simulink model "eVTOL_PX4_2023b"  (R2024b)
settings: Solver=ode4  StartTime=0  StopTime=inf  FixedStep=0.01  RelTol=1e-3
values from neighbouring files (symbols this model uses):
  aDl =     [initdata.mat]
  aDr =     [initdata.mat]
  aDyn =     [initdata.mat]
  Airport = init_airport('PHNL')    [initdata_HIL_eVTOL.m]
  aLat =     [initdata.mat]
  aLon =     [initdata.mat]
  D = Prop.D    [EOM_dt_MC.m]    (also in EOM_get_alf_dt_de_prop_evtol.m = CD * QS)
  dt0 = X(2)    [EOM_get_alf_dt_de_prop_evtol.m]    (also in initdata.mat = 0.258252593971; initdata_HIL_eVTOL.m = EOM_dt_MC)
  EAS0 = TAS0 / EAS2TAS    [initdata_HIL_eVTOL.m]
  FCS = init_FCS    [initdata_HIL_eVTOL.m]
  General = init_layoutdata    [EOM_dt_MC.m]    (also in build_optimized_CA.m; initdata.mat = ; initdata_HIL_eVTOL.m)
  h0 = Con(1)    [EOM_get_alf_dt_de_prop_evtol.m]    (also in initdata.mat = 450; initdata_HIL_eVTOL.m = 50)
  mass = Con(3)    [EOM_get_alf_dt_de_prop_evtol.m]    (also in initdata.mat = 2255.54; initdata_HIL_eVTOL.m = 7)
  Motor = init_motor_evtol    [EOM_dt_MC.m]    (also in initdata.mat = []; initdata_HIL_eVTOL.m)
  Prop = init_propeller_evtol_new    [EOM_dt_MC.m]    (also in initdata_HIL_eVTOL.m)
  R2D = 180/pi    (= 57.2957795131)    [EOM_get_alf_dt_de_prop_evtol.m]    (also in init_FCS.m; init_aerodata_evtol.m; init_airport.m; initdata.mat)
  SAMPLE_TIME = 0.01    [initdata_HIL_eVTOL.m]
  theta0 = -0.0510981441662    [initdata.mat]
undefined symbols (not defined in the file or in its folder): A1, aDa, aDe, aero, asbhl20env, B1, C1, de0, Earth, Environment, INIT_Data, InitData, Kd, Kp, magnitude, Newton, pProp, Raphson, Tc, WGS84
libraries: simulink_extras x63, vrlib x48, sharedtransform x28, simulink x22, slpidlib x20, sharedutil x20, matrix_library x18, aerolibwindfilters x12, aerolibobsolete x8, aerolibasang x8, aerolibatmos2 x6, aerolibfltsims x6
(part 9 of 17)

== system eVTOL_PX4_2023b/Subsystem1/Energy & Power1/thrust_5/Propeller  ==
  rpm : Inport
  V : Inport  Port=2
  rho : Inport  Port=3
  D^5 : Constant  Value=5
  Diameter : Constant  Value=Prop.D
  Divide : Product  Inputs=4
  Divide2 : Product  Inputs=4
  Divide3 : Product  Inputs=**/
  Gain : Gain  Gain=1/60
  Math Function : Math  Operator=magnitude^2  SignedPower=on
  Math Function1 : Math  Operator=magnitude^2  SignedPower=on
  Math Function2 : Math  Operator=magnitude^2  SignedPower=on
  Math Function3 : Math  Operator=pow  SignedPower=on
  Math Function4 : Math  Operator=pow  SignedPower=on
  Scope{,1..4} (5 alike) : Scope
  Subsystem : Subsystem
  get CP : Lookup_n-D  BreakpointsForDimension1=Prop.J  BreakpointsForDimension2=Prop.rpm_grid  IndexSearchMethod=Linear search  BeginIndexSearchUsingPreviousIndexResult=on  Table=Prop.CP  RndMeth=Simplest
      settings: InputPortMap=u0,u1
  get CT : Lookup_n-D  BreakpointsForDimension1=Prop.J  BreakpointsForDimension2=Prop.rpm_grid  IndexSearchMethod=Linear search  BeginIndexSearchUsingPreviousIndexResult=on  Table=Prop.CT  RndMeth=Simplest
      settings: InputPortMap=u0,u1
  "n^3 " : Constant  Value=3
  P_plr (w) : Outport  VectorParamsAs1DForOutWhenUnconnected=off
  T (N) : Outport  Port=2  VectorParamsAs1DForOutWhenUnconnected=off
  eta_p : Outport  Port=3  VectorParamsAs1DForOutWhenUnconnected=off
  wires:
  Divide2/1 -> P_plr (w)/1, Scope/1
  Divide3/1 -> eta_p/1  "eta_p"
  D^5/1 -> Math Function4/2
  Math Function4/1 -> Divide2/4
  "n^3 "/1 -> Math Function3/2
  Math Function3/1 -> Divide2/3
  get CP/1 -> Divide3/3, Divide2/1, Scope3/1
  Subsystem/1(J) -> Scope2/1, get CT/1, Divide3/1, get CP/1
  Divide/1 -> Scope1/1, T (N)/1
  Math Function2/1 -> Divide/4  "D^4"
  Math Function1/1 -> Math Function2/1
  Diameter/1 -> Math Function1/1, Math Function4/1
  Math Function/1 -> Divide/3  "n^2"
  Gain/1 -> Math Function3/1, Math Function/1
  rho/1 -> Divide/2, Divide2/2
  get CT/1 -> Divide3/2, Divide/1, Scope4/1
  V/1 -> Subsystem/1(V)
  rpm/1 -> get CP/2, get CT/2, Gain/1, Subsystem/2(rpm)

== system eVTOL_PX4_2023b/Subsystem1/Energy & Power1/thrust_6/Motor ==
  P_shaft : Inport
  dt : Inport  Port=2
  V : Inport  Port=3
  rpm0 : Inport  Port=4
  rho : Inport  Port=5
  rpm_grid : Inport  Port=6
  Constant : Constant  Value=Motor.Ue
  Constant1 : Constant  Value=Motor.Re
  Constant2 : Constant  Value=Motor.Rm
  Constant3 : Constant  Value=Motor.KE
  Constant4 : Constant  Value=Motor.KT  VectorParams1D=off
  Constant5 : Constant  Value=Motor.Im0
  Constant6 : Constant  Value=0
  D^5 : Constant  Value=5
  Diameter : Constant  Value=Prop.D
  Diameter1 : Constant  Value=Prop.D
  Divide : Product  Inputs=*//
  Ea : Sum  Inputs=+-
  Gain1 : Gain  Gain=30/pi
  Gain2 : Gain  Gain=pi/30
  Gain3 : Gain  Gain=1/60
  Gain4 : Gain  Gain=1/(2*pi)
  Im : Sum
  Integrator : Integrator  InitialConditionSource=external  InitialCondition=600
  Ix : Constant  Value=Prop.Ix
  J : Product  Inputs=*//
  Manual Switch : ManualSwitch
  Math Function : Math  Operator=magnitude^2  SignedPower=on
  Math Function3 : Math  Operator=pow  SignedPower=on
  Math Function4 : Math  Operator=pow  SignedPower=on
  Memory : Memory  InitialCondition=0.1
  N(rpm) : Product  Inputs=*/
  N(rpm)1 : Product  Inputs=/*
  P Scope : Scope  NumInputPorts=2
  P_sp : Product  Inputs=4
  Product1 : Product
  Product2 : Product
  Q : Product  Inputs=4
  RPM 6 : Scope
  Saturation : Saturate  UpperLimit=1047.2  LowerLimit=0.1
  Scope : Scope
  Sum : Sum  Inputs=|+-
  Ueo : Product
  Um : Sum  Inputs=+-
  get CP : Lookup_n-D  BreakpointsForDimension1=Prop.J  BreakpointsForDimension2=Prop.rpm_grid  IndexSearchMethod=Linear search  BeginIndexSearchUsingPreviousIndexResult=on  Table=Prop.CP  RndMeth=Simplest
      settings: InputPortMap=u0,u1
  "n^3 " : Constant  Value=3
  rpm : Outport  VectorParamsAs1DForOutWhenUnconnected=off
  wires:
  Saturation/1 -> Gain1/1, Divide/2
  Gain2/1 -> Integrator/2
  rpm0/1 -> Manual Switch/1
  Gain1/1 -> rpm/1, RPM 6/1  "rpm"
  Sum/1 -> Divide/1  "DP"
  Divide/1 -> Integrator/1  "omega_dot"
  dt/1 -> Ueo/1
  Integrator/1 -> Saturation/1  "omega"
  P_sp/1 -> Scope/1, P Scope/1, Sum/1
  P_shaft/1 -> P Scope/2, Sum/2
  Ix/1 -> Divide/3
  Constant/1 -> Ueo/2
  Ueo/1 -> Um/1
  Product1/1 -> Um/2
  Constant1/1 -> Product1/1
  Um/1 -> Ea/1
  Product2/1 -> Ea/2
  Constant2/1 -> Product2/1
  Ea/1 -> N(rpm)/1
  Constant3/1 -> N(rpm)/2
  Diameter/1 -> J/2
  V/1 -> J/1
  N(rpm)/1 -> Gain3/1
  J/1 -> get CP/1
  rpm_grid/1 -> get CP/2
  Gain4/1 -> Q/2  "CQ"
  D^5/1 -> Math Function4/2
  Diameter1/1 -> Math Function4/1
  Math Function/1 -> Q/3  "n^2"
  Q/1 -> N(rpm)1/2
  Constant4/1 -> N(rpm)1/1
  N(rpm)1/1 -> Im/1
  Constant5/1 -> Im/2
  Im/1 -> Product1/2, Product2/2
  rho/1 -> Q/1, P_sp/3  "rho"
  Math Function3/1 -> P_sp/2  "n^3"
  "n^3 "/1 -> Math Function3/2
  Math Function4/1 -> Q/4, P_sp/4  "D^5"
  get CP/1 -> Gain4/1, P_sp/1  "CP"
  Constant6/1 -> Manual Switch/2
  Manual Switch/1 -> Gain2/1
  Gain3/1 -> Memory/1  "rps"
  Memory/1 -> J/3, Math Function3/1, Math Function/1

== system eVTOL_PX4_2023b/Subsystem1/Energy & Power1/thrust_6/Propeller  ==
  rpm : Inport
  V : Inport  Port=2
  rho : Inport  Port=3
  D^5 : Constant  Value=5
  Diameter : Constant  Value=Prop.D
  Divide : Product  Inputs=4
  Divide2 : Product  Inputs=4
  Divide3 : Product  Inputs=**/
  Gain : Gain  Gain=1/60
  Math Function : Math  Operator=magnitude^2  SignedPower=on
  Math Function1 : Math  Operator=magnitude^2  SignedPower=on
  Math Function2 : Math  Operator=magnitude^2  SignedPower=on
  Math Function3 : Math  Operator=pow  SignedPower=on
  Math Function4 : Math  Operator=pow  SignedPower=on
  Scope{,1..4} (5 alike) : Scope
  Subsystem : Subsystem
  get CP : Lookup_n-D  BreakpointsForDimension1=Prop.J  BreakpointsForDimension2=Prop.rpm_grid  IndexSearchMethod=Linear search  BeginIndexSearchUsingPreviousIndexResult=on  Table=Prop.CP  RndMeth=Simplest
      settings: InputPortMap=u0,u1
  get CT : Lookup_n-D  BreakpointsForDimension1=Prop.J  BreakpointsForDimension2=Prop.rpm_grid  IndexSearchMethod=Linear search  BeginIndexSearchUsingPreviousIndexResult=on  Table=Prop.CT  RndMeth=Simplest
      settings: InputPortMap=u0,u1
  "n^3 " : Constant  Value=3
  P_plr (w) : Outport  VectorParamsAs1DForOutWhenUnconnected=off
  T (N) : Outport  Port=2  VectorParamsAs1DForOutWhenUnconnected=off
  eta_p : Outport  Port=3  VectorParamsAs1DForOutWhenUnconnected=off
  wires:
  Divide2/1 -> P_plr (w)/1, Scope/1
  Divide3/1 -> eta_p/1  "eta_p"
  D^5/1 -> Math Function4/2
  Math Function4/1 -> Divide2/4
  "n^3 "/1 -> Math Function3/2
  Math Function3/1 -> Divide2/3
  get CP/1 -> Divide3/3, Divide2/1, Scope3/1
  Subsystem/1(J) -> Scope2/1, get CT/1, Divide3/1, get CP/1
  Divide/1 -> Scope1/1, T (N)/1
  Math Function2/1 -> Divide/4  "D^4"
  Math Function1/1 -> Math Function2/1
  Diameter/1 -> Math Function1/1, Math Function4/1
  Math Function/1 -> Divide/3  "n^2"
  Gain/1 -> Math Function3/1, Math Function/1
  rho/1 -> Divide/2, Divide2/2
  get CT/1 -> Divide3/2, Divide/1, Scope4/1
  V/1 -> Subsystem/1(V)
  rpm/1 -> get CP/2, get CT/2, Gain/1, Subsystem/2(rpm)

== system eVTOL_PX4_2023b/Subsystem1/Environment/Wind Models/Dryden Wind Turbulence Model (Continuous (+q -r)) ==
  Altitude : Inport  Unit=m
  Airspeed : Inport  Port=2  Unit=m/s
  DCM : Inport  Port=3  Unit=1  PortDimensions=[3 3]
  (u,v,w) : Selector  InputPortWidth=4  IndexOptions=Index vector (dialog)  Indices=[1 2 3]  OutputSizes=1
  Angle Conversion : Subsystem
  Bus Creator : BusCreator  Inputs=3
  Cast : DataTypeConversion  SaturateOnIntegerOverflow=off  RndMeth=Floor
  Cast To Double{,1..4} (5 alike) : DataTypeConversion  OutDataTypeStr=double  SaturateOnIntegerOverflow=off  RndMeth=Floor
  Disallow CGS : UnitConfiguration  UnitSystemsStr=English,SI,SI (extended)  AllowAllUnitSystems=off
  Filters on angular rates : Subsystem  mask(Angular Rates){}
  Filters on velocities : aerolibwindfilters/Dryden Continuous Filters  SystemSampleTime=-1  VariantActivationTime=update diagram  AllowFlexibleInterface=on  Latency=0  AutoFrameSizeCalculation=off
  Length Conversion : Subsystem
  Length Conversion1 : Subsystem
  Mux : Mux  Inputs=3
  Mux1 : Mux  Inputs=3
  RMS turbulence intensities : Subsystem
  Select angular rates : Subsystem
  Select velocities : Subsystem
  Turbulence scale lengths : Subsystem
  Unit Conversion : UnitConversion  OutputType=Inherit: Inherit via back propagation
  Velocity Conversion : Subsystem
  Velocity Conversion2 : Subsystem
  White Noise : aerolibcommonsys/Tunable White Noise  pwr=[1 1 1 1]*pi  Ts=ts  seed=Seed
  Wind direction : Constant  Value=Wdeg
  Windspeed at 20ft (6m) : Constant  Value=W20
  Wingspan : Constant  Value=Wingspan
  p : Selector  InputPortWidth=4  IndexOptions=Index vector (dialog)  Indices=[4]  OutputSizes=1
  ug,vg,wg : Outport  Unit=m/s  VectorParamsAs1DForOutWhenUnconnected=off
  pg,qg,rg : Outport  Port=2  VectorParamsAs1DForOutWhenUnconnected=off
  wires:
  Cast To Double4/1 -> Velocity Conversion/1(in)
  Airspeed/1 -> Cast To Double4/1
  Cast To Double3/1 -> Length Conversion1/1(in)
  Wingspan/1 -> Cast To Double3/1
  Cast To Double2/1 -> Length Conversion/1(in)
  Cast To Double1/1 -> Angle Conversion/1(in)
  Cast To Double/1 -> Bus Creator/1  "DCM"
  Mux1/1 -> Cast/1
  Cast/1 -> pg,qg,rg/1
  (u,v,w)/1 -> Filters on velocities/1
  Unit Conversion/1 -> ug,vg,wg/1
  Velocity Conversion/1(out) -> Filters on angular rates/3(V), Filters on velocities/8
  Angle Conversion/1(out) -> Bus Creator/2  "Wdeg"
  Length Conversion1/1(out) -> Filters on angular rates/7(wingspan)
  Bus Creator/1 -> Select angular rates/4("DCM, altitude, Wdeg"), Select velocities/1("DCM, altitude, Wdeg")
  DCM/1 -> Cast To Double/1  "DCM"
  Wind direction/1 -> Cast To Double1/1
  Select angular rates/3(rgw) -> Mux1/3
  Select angular rates/2(qgw) -> Mux1/2
  Select angular rates/1(pgw) -> Mux1/1
  Select velocities/3(wgw) -> Mux/3
  Select velocities/2(vgw) -> Mux/2
  Select velocities/1(ugw) -> Mux/1
  Velocity Conversion2/1(out) -> RMS turbulence intensities/2(Windspeed at 20ft (6m))
  Windspeed at 20ft (6m)/1 -> Velocity Conversion2/1(in)
  RMS turbulence intensities/2(sigma_vg) -> Filters on velocities/6
  Filters on velocities/3 -> Filters on angular rates/2(wg), Select velocities/4(wgw_h&l)  "wgw"
  Filters on velocities/2 -> Filters on angular rates/1(vg), Select velocities/3(vgw_h&l)  "vgw"
  RMS turbulence intensities/1("sigma_ug ") -> Filters on velocities/5
  Filters on velocities/1 -> Select velocities/2(ugw_h&l)  "ugw"
  Filters on angular rates/3(rgw) -> Select angular rates/3(rgw_h&l)  "rgw"
  Filters on angular rates/2(qgw) -> Select angular rates/2(qgw_h&l)  "qgw"
  Filters on angular rates/1(pgw) -> Select angular rates/1(pgw_h&l)  "pgw"
  RMS turbulence intensities/3(sigma_wg) -> Filters on angular rates/5(sigma_w), Filters on velocities/7
  Turbulence scale lengths/3(L_wg) -> Filters on angular rates/4(Lw), Filters on velocities/4
  Turbulence scale lengths/1(L_ug) -> Filters on velocities/2
  Altitude/1 -> Cast To Double2/1
  Mux/1 -> Unit Conversion/1
  White Noise/1 -> (u,v,w)/1, p/1
  p/1 -> Filters on angular rates/6(Noise)
  Length Conversion/1(out) -> Bus Creator/3, RMS turbulence intensities/1(Altitude), Turbulence scale lengths/1(Altitude)  "altitude"
  Turbulence scale lengths/2(L_vg) -> Filters on velocities/3

== system eVTOL_PX4_2023b/Subsystem1/Environment1/Wind Models/Dryden Wind Turbulence Model (Continuous (+q -r)) ==
  Altitude : Inport  Unit=m
  Airspeed : Inport  Port=2  Unit=m/s
  DCM : Inport  Port=3  Unit=1  PortDimensions=[3 3]
  (u,v,w) : Selector  InputPortWidth=4  IndexOptions=Index vector (dialog)  Indices=[1 2 3]  OutputSizes=1
  Angle Conversion : Subsystem
  Bus Creator : BusCreator  Inputs=3
  Cast : DataTypeConversion  SaturateOnIntegerOverflow=off  RndMeth=Floor
  Cast To Double{,1..4} (5 alike) : DataTypeConversion  OutDataTypeStr=double  SaturateOnIntegerOverflow=off  RndMeth=Floor
  Disallow CGS : UnitConfiguration  UnitSystemsStr=English,SI,SI (extended)  AllowAllUnitSystems=off
  Filters on angular rates : Subsystem  mask(Angular Rates){}
  Filters on velocities : aerolibwindfilters/Dryden Continuous Filters  SystemSampleTime=-1  VariantActivationTime=update diagram  AllowFlexibleInterface=on  Latency=0  AutoFrameSizeCalculation=off
  Length Conversion : Subsystem
  Length Conversion1 : Subsystem
  Mux : Mux  Inputs=3
  Mux1 : Mux  Inputs=3
  RMS turbulence intensities : Subsystem
  Select angular rates : Subsystem
  Select velocities : Subsystem
  Turbulence scale lengths : Subsystem
  Unit Conversion : UnitConversion  OutputType=Inherit: Inherit via back propagation
  Velocity Conversion : Subsystem
  Velocity Conversion2 : Subsystem
  White Noise : aerolibcommonsys/Tunable White Noise  pwr=[1 1 1 1]*pi  Ts=ts  seed=Seed
  Wind direction : Constant  Value=Wdeg
  Windspeed at 20ft (6m) : Constant  Value=W20
  Wingspan : Constant  Value=Wingspan
  p : Selector  InputPortWidth=4  IndexOptions=Index vector (dialog)  Indices=[4]  OutputSizes=1
  ug,vg,wg : Outport  Unit=m/s  VectorParamsAs1DForOutWhenUnconnected=off
  pg,qg,rg : Outport  Port=2  VectorParamsAs1DForOutWhenUnconnected=off
  wires:
  Cast To Double4/1 -> Velocity Conversion/1(in)
  Airspeed/1 -> Cast To Double4/1
  Cast To Double3/1 -> Length Conversion1/1(in)
  Wingspan/1 -> Cast To Double3/1
  Cast To Double2/1 -> Length Conversion/1(in)
  Cast To Double1/1 -> Angle Conversion/1(in)
  Cast To Double/1 -> Bus Creator/1  "DCM"
  Mux1/1 -> Cast/1
  Cast/1 -> pg,qg,rg/1
  (u,v,w)/1 -> Filters on velocities/1
  Unit Conversion/1 -> ug,vg,wg/1
  Velocity Conversion/1(out) -> Filters on angular rates/3(V), Filters on velocities/8
  Angle Conversion/1(out) -> Bus Creator/2  "Wdeg"
  Length Conversion1/1(out) -> Filters on angular rates/7(wingspan)
  Bus Creator/1 -> Select angular rates/4("DCM, altitude, Wdeg"), Select velocities/1("DCM, altitude, Wdeg")
  DCM/1 -> Cast To Double/1  "DCM"
  Wind direction/1 -> Cast To Double1/1
  Select angular rates/3(rgw) -> Mux1/3
  Select angular rates/2(qgw) -> Mux1/2
  Select angular rates/1(pgw) -> Mux1/1
  Select velocities/3(wgw) -> Mux/3
  Select velocities/2(vgw) -> Mux/2
  Select velocities/1(ugw) -> Mux/1
  Velocity Conversion2/1(out) -> RMS turbulence intensities/2(Windspeed at 20ft (6m))
  Windspeed at 20ft (6m)/1 -> Velocity Conversion2/1(in)
  RMS turbulence intensities/2(sigma_vg) -> Filters on velocities/6
  Filters on velocities/3 -> Filters on angular rates/2(wg), Select velocities/4(wgw_h&l)  "wgw"
  Filters on velocities/2 -> Filters on angular rates/1(vg), Select velocities/3(vgw_h&l)  "vgw"
  RMS turbulence intensities/1("sigma_ug ") -> Filters on velocities/5
  Filters on velocities/1 -> Select velocities/2(ugw_h&l)  "ugw"
  Filters on angular rates/3(rgw) -> Select angular rates/3(rgw_h&l)  "rgw"
  Filters on angular rates/2(qgw) -> Select angular rates/2(qgw_h&l)  "qgw"
  Filters on angular rates/1(pgw) -> Select angular rates/1(pgw_h&l)  "pgw"
  RMS turbulence intensities/3(sigma_wg) -> Filters on angular rates/5(sigma_w), Filters on velocities/7
  Turbulence scale lengths/3(L_wg) -> Filters on angular rates/4(Lw), Filters on velocities/4
  Turbulence scale lengths/1(L_ug) -> Filters on velocities/2
  Altitude/1 -> Cast To Double2/1
  Mux/1 -> Unit Conversion/1
  White Noise/1 -> (u,v,w)/1, p/1
  p/1 -> Filters on angular rates/6(Noise)
  Length Conversion/1(out) -> Bus Creator/3, RMS turbulence intensities/1(Altitude), Turbulence scale lengths/1(Altitude)  "altitude"
  Turbulence scale lengths/2(L_vg) -> Filters on velocities/3

== system eVTOL_PX4_2023b/Subsystem1/airframe/Flight Conditions/Incidence, Sideslip, & Airspeed ==
  Vb : Inport
  Airspeed : Math  Operator=sqrt  SignedPower=on
  Incidence : Trigonometry  Operator=atan2
  Product : Product  Inputs=*/  SaturateOnIntegerOverflow=on  OutDataTypeStr=Inherit: Same as first input
  Sideslip : Trigonometry  Operator=asin
  Subsystem : Subsystem
  Subsystem1 : Subsystem
  dot : Subsystem
  Alpha : Outport  InitialOutput=0  VectorParamsAs1DForOutWhenUnconnected=off
  Beta : Outport  Port=2  InitialOutput=0  VectorParamsAs1DForOutWhenUnconnected=off
  V : Outport  Port=3  InitialOutput=0  VectorParamsAs1DForOutWhenUnconnected=off
  wires:
  Product/1 -> Sideslip/1
  Subsystem/1(w) -> Incidence/1
  Subsystem/2(U) -> Incidence/2
  dot/1(dot) -> Airspeed/1
  Airspeed/1 -> Product/2, V/1
  Incidence/1 -> Alpha/1
  Vb/1 -> Subsystem/1(V), dot/1(Vb), Subsystem1/1(V)
  Sideslip/1 -> Beta/1
  Subsystem1/1(v) -> Product/1

== system eVTOL_PX4_2023b/Subsystem1/airframe/Flight Conditions/Subsystem ==
  <Ve> : Inport
  Atan1 : Trigonometry  Operator=atan2
  Atan2 : Trigonometry  Operator=atan2
  Dot Product : DotProduct  OutDataTypeStr=Inherit: Inherit via internal rule
  Gain : Gain  Gain=-1
  Selector : Selector  InputPortWidth=3  IndexOptions=Index vector (dialog)  Indices=1  OutputSizes=1
  Selector1 : Selector  InputPortWidth=3  IndexOptions=Index vector (dialog)  Indices=2  OutputSizes=1
  Selector2 : Selector  InputPortWidth=3  IndexOptions=Index vector (dialog)  Indices=3  OutputSizes=1
  Sqrt : Sqrt
  gamma : Outport  InitialOutput=0  VectorParamsAs1DForOutWhenUnconnected=off
  chi : Outport  Port=2  InitialOutput=0  VectorParamsAs1DForOutWhenUnconnected=off
  V : Outport  Port=3  InitialOutput=0  VectorParamsAs1DForOutWhenUnconnected=off
  wires:
  Selector/1 -> Atan1/2
  Selector2/1 -> Gain/1
  <Ve>/1 -> Selector/1, Selector1/1, Selector2/1, Dot Product/1, Dot Product/2
  Atan2/1 -> gamma/1
  Selector1/1 -> Atan1/1
  Sqrt/1 -> V/1, Atan2/2
  Atan1/1 -> chi/1
  Gain/1 -> Atan2/1
  Dot Product/1 -> Sqrt/1

== system eVTOL_PX4_2023b/Subsystem1/airframe/force moment/Gear&FM in body axis ==
  PlantData : Inport
  Add1 : Sum  Inputs=++++
  Add2 : Sum  Inputs=++++
  Constant1 : Constant  Value=0
  Constant6 : Constant  Value=0
  F 4 gear : Scope  NumInputPorts=4
  F&M  Front Gear Left : Subsystem
  F&M  Front Gear Right : Subsystem
  F&M  Main Gear Left : Subsystem
  F&M  Main Gear Right : Subsystem
  M 4 gear : Scope  NumInputPorts=4
  F_Gear : Outport  VectorParamsAs1DForOutWhenUnconnected=off
  M_Gear : Outport  Port=2  VectorParamsAs1DForOutWhenUnconnected=off
  wires:
  PlantData/1 -> F&M  Main Gear Right/1(PlantData), F&M  Main Gear Left/1(PlantData), F&M  Front Gear Right/1(PlantData), F&M  Front Gear Left/1(PlantData)
  F&M  Front Gear Left/2(M_fgl) -> M 4 gear/1, Add2/1
  F&M  Front Gear Left/1(F_fgl) -> F 4 gear/1, Add1/1
  F&M  Front Gear Right/1(F_fgl) -> F 4 gear/2, Add1/2
  F&M  Main Gear Left/1(F_fgl) -> F 4 gear/3, Add1/3
  F&M  Main Gear Right/1(F_fgl) -> F 4 gear/4, Add1/4
  Add1/1 -> F_Gear/1
  F&M  Front Gear Right/2(M_fgl) -> M 4 gear/2, Add2/2
  F&M  Main Gear Left/2(M_fgl) -> M 4 gear/3, Add2/3
  F&M  Main Gear Right/2(M_fgl) -> M 4 gear/4, Add2/4
  Add2/1 -> M_Gear/1
  Constant6/1 -> F&M  Main Gear Left/2(dg)
  Constant1/1 -> F&M  Main Gear Right/2(dg)

== system eVTOL_PX4_2023b/Subsystem1/airframe/force moment/Gear&FM in body axis1 ==
  PlantData : Inport
  Add1 : Sum  Inputs=++++
  Add2 : Sum  Inputs=++++
  Constant1 : Constant  Value=0
  Constant6 : Constant  Value=0
  F 4 gear : Scope  NumInputPorts=4
  F&M  Front Gear Left : Subsystem
  F&M  Front Gear Right : Subsystem
  F&M  Main Gear Left : Subsystem
  F&M  Main Gear Right : Subsystem
  M 4 gear : Scope  NumInputPorts=4
  F_Gear : Outport  VectorParamsAs1DForOutWhenUnconnected=off
  M_Gear : Outport  Port=2  VectorParamsAs1DForOutWhenUnconnected=off
  wires:
  PlantData/1 -> F&M  Main Gear Right/1(PlantData), F&M  Main Gear Left/1(PlantData), F&M  Front Gear Right/1(PlantData), F&M  Front Gear Left/1(PlantData)
  F&M  Front Gear Left/2(M_fgl) -> M 4 gear/1, Add2/1
  F&M  Front Gear Left/1(F_fgl) -> F 4 gear/1, Add1/1
  F&M  Front Gear Right/1(F_fgl) -> F 4 gear/2, Add1/2
  F&M  Main Gear Left/1(F_fgl) -> F 4 gear/3, Add1/3
  F&M  Main Gear Right/1(F_fgl) -> F 4 gear/4, Add1/4
  Add1/1 -> F_Gear/1
  F&M  Front Gear Right/2(M_fgl) -> M 4 gear/2, Add2/2
  F&M  Main Gear Left/2(M_fgl) -> M 4 gear/3, Add2/3
  F&M  Main Gear Right/2(M_fgl) -> M 4 gear/4, Add2/4
  Add2/1 -> M_Gear/1
  Constant6/1 -> F&M  Main Gear Left/2(dg)
  Constant1/1 -> F&M  Main Gear Right/2(dg)

== system eVTOL_PX4_2023b/Subsystem1/airframe/force moment/Thrust&M in body axis ==
  prop : Inport
  3x3 Cross Product{,1..5} (6 alike) : sharedutil/3x3 Cross Product  aMode=aMode
  Bus Selector1 : BusSelector  OutputSignals=T_1,T_2,T_3,T_4,T_5,T_6,Q
  Constant1 : Constant  Value=General.pos_plr3
  Constant2 : Constant  Value=General.pos_plr4
  Constant3 : Constant  Value=General.pos_plr5
  Constant4 : Constant  Value=General.pos_plr1
  Constant5 : Constant  Value=General.pos_plr6
  Constant6 : Constant  Value=General.pos_plr2
  Display3 : Display
  Scope2 : Scope
  Sum2 : Sum  Inputs=++++++
  Sum3 : Sum  Inputs=++++++
  Sum4 : Sum  Inputs=++|
  T MC : Scope  NumInputPorts=6
  f_T : Outport  VectorParamsAs1DForOutWhenUnconnected=off
  m_T : Outport  Port=2  VectorParamsAs1DForOutWhenUnconnected=off
  wires:
  prop/1 -> Bus Selector1/1
  Constant4/1 -> 3x3 Cross Product/1
  Constant6/1 -> 3x3 Cross Product1/1
  Constant1/1 -> 3x3 Cross Product2/1
  Constant2/1 -> 3x3 Cross Product3/1
  Bus Selector1/1 -> T MC/1, [T_1]  "<T_1>"
  Bus Selector1/2 -> [T_2], T MC/2  "<T_2>"
  Bus Selector1/3 -> [T_3], T MC/3  "<T_3>"
  Bus Selector1/4 -> [T_4], T MC/4  "<T_4>"
  [T_1] -> 3x3 Cross Product/2
  [T_2] -> 3x3 Cross Product1/2
  [T_3] -> 3x3 Cross Product2/2
  [T_4] -> 3x3 Cross Product3/2
  [T_1] -> Sum2/1
  [T_2] -> Sum2/2
  [T_3] -> Sum2/3
  [T_4] -> Sum2/4
  3x3 Cross Product/1 -> Sum3/1
  3x3 Cross Product1/1 -> Sum3/2
  3x3 Cross Product2/1 -> Sum3/3
  3x3 Cross Product3/1 -> Sum3/4
  Sum2/1 -> f_T/1, Scope2/1, Display3/1  "T"
  Sum3/1 -> Sum4/2
  Bus Selector1/5 -> [T_5], T MC/5  "<T_5>"
  Sum4/1 -> m_T/1
  [Q] -> Sum4/1
  Bus Selector1/6 -> T MC/6, [T_6]  "<T_6>"
  Bus Selector1/7 -> [Q]  "<Q>"
  [T_5] -> Sum2/5
  [T_6] -> Sum2/6
  [T_5] -> 3x3 Cross Product4/2
  3x3 Cross Product4/1 -> Sum3/5
  Constant3/1 -> 3x3 Cross Product4/1
  [T_6] -> 3x3 Cross Product5/2
  3x3 Cross Product5/1 -> Sum3/6
  Constant5/1 -> 3x3 Cross Product5/1

== system eVTOL_PX4_2023b/Subsystem1/airframe/force moment/aero F&M in body axis ==
  PlantData : Inport
  Act_surface : Inport  Port=2
  Aerodynamic Coefficients : Subsystem  AncestorBlock=asbhl20vehicle/Vehicle/Aerodynamic/Aerodynamic Coefficients
      settings: LibrarySourceBlock=|
      | asbhl20vehicle/Vehicle/Aerodynamic/Aerodynamic
      | Coefficients
  "Aerodynamic Forces and Moments " : aerolibadyn/Aerodynamic Forces and Moments   inputAxes=Body  outputForceAxes=Body  outputMomentAxes=Body  S=General.Sw  b=General.b  cbar=General.MAC
  Center of Gravity : Constant  Value=[0 0 0]  SampleTime=0
  Center of Pressure : Constant  Value=[0 0 0]  SampleTime=0
  Constant : Constant
  Constant1 : Constant  Commented=on
  Mux1 : Mux  Inputs=2
  PlantBus : BusSelector  OutputSignals=Vb,alpha,beta,Va,pqr,alphaDot,mach
  PlantBus1 : BusSelector  OutputSignals=Q
  PlantData_1 : InportShadow
  Product : Product
  Product1 : Product
  Scope1 : Scope  Commented=on
  Scope2 : Scope
  Scope3 : Scope
  Scope4 : Scope  Commented=on
  Selector : Selector  Commented=on  InputPortWidth=3  IndexOptions=Index vector (dialog)  Indices=1  OutputSizes=1
  Switch : Switch  Commented=on  Criteria=u2 > Threshold  Threshold=3  SaturateOnIntegerOverflow=off  InputSameDT=off
  nonunit value : Subsystem
  Fb (X Y Z) : Outport  VectorParamsAs1DForOutWhenUnconnected=off
  M (L M N) : Outport  Port=2  VectorParamsAs1DForOutWhenUnconnected=off
  wires:
  "Aerodynamic Forces and Moments "/1 -> Product/1, Scope2/1
  "Aerodynamic Forces and Moments "/2 -> Product1/1, Scope3/1
  PlantData/1 -> PlantBus/1
  Act_surface/1 -> Aerodynamic Coefficients/5(Act_surface)
  PlantBus/2 -> Mux1/1  "<alpha>"
  PlantBus/3 -> Mux1/2  "<beta>"
  PlantBus/5 -> nonunit value/2(pqr)  "<pqr>"
  Center of Gravity/1 -> "Aerodynamic Forces and Moments "/3
  Center of Pressure/1 -> "Aerodynamic Forces and Moments "/4
  PlantBus1/1 -> "Aerodynamic Forces and Moments "/2  "<Q>"
  PlantData_1/1 -> PlantBus1/1
  PlantBus/6 -> nonunit value/3(alphaDot)  "<alphaDot>"
  PlantBus/4 -> nonunit value/1(V)  "<Va>"
  Constant1/1 -> Switch/1
  Constant/1 -> [Aero_SW]
  Switch/1 -> Scope1/1
  Product/1 -> Fb (X Y Z)/1
  Product1/1 -> M (L M N)/1
  [Aero_SW] -> Product/2
  [Aero_SW] -> Product1/2
  PlantBus/1 -> Selector/1  "<Vb>"
  Selector/1 -> Switch/2, Scope4/1  "Vb_x"
  Mux1/1 -> Aerodynamic Coefficients/1(Incid)
  nonunit value/1(pqr_n) -> Aerodynamic Coefficients/3(pqrn)
  nonunit value/2(alphaDot_n) -> Aerodynamic Coefficients/4(alphaDot_n)
  Aerodynamic Coefficients/1(Coeff) -> "Aerodynamic Forces and Moments "/1
  PlantBus/7 -> Aerodynamic Coefficients/2(mach)  "<mach>"

== system eVTOL_PX4_2023b/Subsystem1/airframe/force moment/gravity in body axis ==
  PlantData : Inport
  EnvmData : Inport  Port=2
  Bus Selector1 : BusSelector  OutputSignals=DCM_be,mass
  Bus Selector2 : BusSelector  OutputSignals=g
  G in body axis : Product  Multiplication=Matrix(*)  RndMeth=Zero
  Gain1 : Gain  Gain=[0; 0; 1]
  Product : Product  RndMeth=Zero
  Fb : Outport  VectorParamsAs1DForOutWhenUnconnected=off
  wires:
  Bus Selector1/1 -> G in body axis/1  "<DCM_be>"
  Gain1/1 -> G in body axis/2
  Bus Selector1/2 -> Product/1  "<mass>"
  Bus Selector2/1 -> Product/2  "<g>"
  Product/1 -> Gain1/1  "mg"
  PlantData/1 -> Bus Selector1/1
  G in body axis/1 -> Fb/1
  EnvmData/1 -> Bus Selector2/1

== system eVTOL_PX4_2023b/Subsystem1/airframe1/Flight Conditions/Incidence, Sideslip, & Airspeed ==
  Vb : Inport
  Airspeed : Math  Operator=sqrt  SignedPower=on
  Incidence : Trigonometry  Operator=atan2
  Product : Product  Inputs=*/  SaturateOnIntegerOverflow=on  OutDataTypeStr=Inherit: Same as first input
  Sideslip : Trigonometry  Operator=asin
  Subsystem : Subsystem
  Subsystem1 : Subsystem
  dot : Subsystem
  Alpha : Outport  InitialOutput=0  VectorParamsAs1DForOutWhenUnconnected=off
  Beta : Outport  Port=2  InitialOutput=0  VectorParamsAs1DForOutWhenUnconnected=off
  V : Outport  Port=3  InitialOutput=0  VectorParamsAs1DForOutWhenUnconnected=off
  wires:
  Product/1 -> Sideslip/1
  Subsystem/1(w) -> Incidence/1
  Subsystem/2(U) -> Incidence/2
  dot/1(dot) -> Airspeed/1
  Airspeed/1 -> Product/2, V/1
  Incidence/1 -> Alpha/1
  Vb/1 -> Subsystem/1(V), dot/1(Vb), Subsystem1/1(V)
  Sideslip/1 -> Beta/1
  Subsystem1/1(v) -> Product/1

== system eVTOL_PX4_2023b/Subsystem1/airframe1/Flight Conditions/Subsystem ==
  <Ve> : Inport
  Atan1 : Trigonometry  Operator=atan2
  Atan2 : Trigonometry  Operator=atan2
  Dot Product : DotProduct  OutDataTypeStr=Inherit: Inherit via internal rule
  Gain : Gain  Gain=-1
  Selector : Selector  InputPortWidth=3  IndexOptions=Index vector (dialog)  Indices=1  OutputSizes=1
  Selector1 : Selector  InputPortWidth=3  IndexOptions=Index vector (dialog)  Indices=2  OutputSizes=1
  Selector2 : Selector  InputPortWidth=3  IndexOptions=Index vector (dialog)  Indices=3  OutputSizes=1
  Sqrt : Sqrt
  gamma : Outport  InitialOutput=0  VectorParamsAs1DForOutWhenUnconnected=off
  chi : Outport  Port=2  InitialOutput=0  VectorParamsAs1DForOutWhenUnconnected=off
  V : Outport  Port=3  InitialOutput=0  VectorParamsAs1DForOutWhenUnconnected=off
  wires:
  Selector/1 -> Atan1/2
  Selector2/1 -> Gain/1
  <Ve>/1 -> Selector/1, Selector1/1, Selector2/1, Dot Product/1, Dot Product/2
  Atan2/1 -> gamma/1
  Selector1/1 -> Atan1/1
  Sqrt/1 -> V/1, Atan2/2
  Atan1/1 -> chi/1
  Gain/1 -> Atan2/1
  Dot Product/1 -> Sqrt/1

== system eVTOL_PX4_2023b/Subsystem1/airframe1/force moment/Gear&FM in body axis ==
  PlantData : Inport
  Add1 : Sum  Inputs=++++
  Add2 : Sum  Inputs=++++
  Constant1 : Constant  Value=0
  Constant6 : Constant  Value=0
  F 4 gear : Scope  NumInputPorts=4
  F&M  Front Gear Left : Subsystem
  F&M  Front Gear Right : Subsystem
  F&M  Main Gear Left : Subsystem
  F&M  Main Gear Right : Subsystem
  M 4 gear : Scope  NumInputPorts=4
  F_Gear : Outport  VectorParamsAs1DForOutWhenUnconnected=off
  M_Gear : Outport  Port=2  VectorParamsAs1DForOutWhenUnconnected=off
  wires:
  PlantData/1 -> F&M  Main Gear Right/1(PlantData), F&M  Main Gear Left/1(PlantData), F&M  Front Gear Right/1(PlantData), F&M  Front Gear Left/1(PlantData)
  F&M  Front Gear Left/2(M_fgl) -> M 4 gear/1, Add2/1
  F&M  Front Gear Left/1(F_fgl) -> F 4 gear/1, Add1/1
  F&M  Front Gear Right/1(F_fgl) -> F 4 gear/2, Add1/2
  F&M  Main Gear Left/1(F_fgl) -> F 4 gear/3, Add1/3
  F&M  Main Gear Right/1(F_fgl) -> F 4 gear/4, Add1/4
  Add1/1 -> F_Gear/1
  F&M  Front Gear Right/2(M_fgl) -> M 4 gear/2, Add2/2
  F&M  Main Gear Left/2(M_fgl) -> M 4 gear/3, Add2/3
  F&M  Main Gear Right/2(M_fgl) -> M 4 gear/4, Add2/4
  Add2/1 -> M_Gear/1
  Constant6/1 -> F&M  Main Gear Left/2(dg)
  Constant1/1 -> F&M  Main Gear Right/2(dg)

== system eVTOL_PX4_2023b/Subsystem1/airframe1/force moment/Gear&FM in body axis1 ==
  PlantData : Inport
  Add1 : Sum  Inputs=++++
  Add2 : Sum  Inputs=++++
  Constant1 : Constant  Value=0
  Constant6 : Constant  Value=0
  F 4 gear : Scope  NumInputPorts=4
  F&M  Front Gear Left : Subsystem
  F&M  Front Gear Right : Subsystem
  F&M  Main Gear Left : Subsystem
  F&M  Main Gear Right : Subsystem
  Gain : Gain  Gain=0.005
  Gain1 : Gain  Gain=0.005
  M 4 gear : Scope  NumInputPorts=4
  F_Gear : Outport  VectorParamsAs1DForOutWhenUnconnected=off
  M_Gear : Outport  Port=2  VectorParamsAs1DForOutWhenUnconnected=off
  wires:
  PlantData/1 -> F&M  Main Gear Right/1(PlantData), F&M  Main Gear Left/1(PlantData), F&M  Front Gear Right/1(PlantData), F&M  Front Gear Left/1(PlantData)
  F&M  Front Gear Left/2(M_fgl) -> M 4 gear/1, Add2/1
  F&M  Front Gear Left/1(F_fgl) -> F 4 gear/1, Add1/1
  F&M  Front Gear Right/1(F_fgl) -> F 4 gear/2, Add1/2
  F&M  Main Gear Left/1(F_fgl) -> F 4 gear/3, Add1/3
  F&M  Main Gear Right/1(F_fgl) -> F 4 gear/4, Add1/4
  F&M  Front Gear Right/2(M_fgl) -> M 4 gear/2, Add2/2
  F&M  Main Gear Left/2(M_fgl) -> M 4 gear/3, Add2/3
  F&M  Main Gear Right/2(M_fgl) -> M 4 gear/4, Add2/4
  Constant6/1 -> F&M  Main Gear Left/2(dg)
  Constant1/1 -> F&M  Main Gear Right/2(dg)
  Add1/1 -> Gain/1
  Gain/1 -> F_Gear/1
  Add2/1 -> Gain1/1
  Gain1/1 -> M_Gear/1

== system eVTOL_PX4_2023b/Subsystem1/airframe1/force moment/Thrust&M in body axis ==
  prop : Inport
  3x3 Cross Product{,1..5} (6 alike) : sharedutil/3x3 Cross Product  aMode=aMode
  Bus Selector1 : BusSelector  OutputSignals=T_1,T_2,T_3,T_4,T_5,T_6,Q
  Constant1 : Constant  Value=General.pos_plr3
  Constant2 : Constant  Value=General.pos_plr4
  Constant3 : Constant  Value=General.pos_plr5
  Constant4 : Constant  Value=General.pos_plr1
  Constant5 : Constant  Value=General.pos_plr6
  Constant6 : Constant  Value=General.pos_plr2
  Display3 : Display
  Scope2 : Scope
  Sum2 : Sum  Inputs=++++++
  Sum3 : Sum  Inputs=++++++
  Sum4 : Sum  Inputs=++|
  T MC : Scope  NumInputPorts=6
  f_T : Outport  VectorParamsAs1DForOutWhenUnconnected=off
  m_T : Outport  Port=2  VectorParamsAs1DForOutWhenUnconnected=off
  wires:
  prop/1 -> Bus Selector1/1
  Constant4/1 -> 3x3 Cross Product/1
  Constant6/1 -> 3x3 Cross Product1/1
  Constant1/1 -> 3x3 Cross Product2/1
  Constant2/1 -> 3x3 Cross Product3/1
  Bus Selector1/1 -> T MC/1, [T_1]  "<T_1>"
  Bus Selector1/2 -> [T_2], T MC/2  "<T_2>"
  Bus Selector1/3 -> [T_3], T MC/3  "<T_3>"
  Bus Selector1/4 -> [T_4], T MC/4  "<T_4>"
  [T_1] -> 3x3 Cross Product/2
  [T_2] -> 3x3 Cross Product1/2
  [T_3] -> 3x3 Cross Product2/2
  [T_4] -> 3x3 Cross Product3/2
  [T_1] -> Sum2/1
  [T_2] -> Sum2/2
  [T_3] -> Sum2/3
  [T_4] -> Sum2/4
  3x3 Cross Product/1 -> Sum3/1
  3x3 Cross Product1/1 -> Sum3/2
  3x3 Cross Product2/1 -> Sum3/3
  3x3 Cross Product3/1 -> Sum3/4
  Sum2/1 -> f_T/1, Scope2/1, Display3/1  "T"
  Sum3/1 -> Sum4/2
  Bus Selector1/5 -> [T_5], T MC/5  "<T_5>"
  Sum4/1 -> m_T/1
  [Q] -> Sum4/1
  Bus Selector1/6 -> T MC/6, [T_6]  "<T_6>"
  Bus Selector1/7 -> [Q]  "<Q>"
  [T_5] -> Sum2/5
  [T_6] -> Sum2/6
  [T_5] -> 3x3 Cross Product4/2
  3x3 Cross Product4/1 -> Sum3/5
  Constant3/1 -> 3x3 Cross Product4/1
  [T_6] -> 3x3 Cross Product5/2
  3x3 Cross Product5/1 -> Sum3/6
  Constant5/1 -> 3x3 Cross Product5/1

== system eVTOL_PX4_2023b/Subsystem1/airframe1/force moment/aero F&M in body axis ==
  PlantData : Inport
  Act_surface : Inport  Port=2
  Aerodynamic Coefficients : Subsystem  AncestorBlock=asbhl20vehicle/Vehicle/Aerodynamic/Aerodynamic Coefficients
      settings: LibrarySourceBlock=|
      | asbhl20vehicle/Vehicle/Aerodynamic/Aerodynamic
      | Coefficients
  "Aerodynamic Forces and Moments " : aerolibadyn/Aerodynamic Forces and Moments   inputAxes=Body  outputForceAxes=Body  outputMomentAxes=Body  S=General.Sw  b=General.b  cbar=General.MAC
  Center of Gravity : Constant  Value=[0 0 0]  SampleTime=0
  Center of Pressure : Constant  Value=[0 0 0]  SampleTime=0
  Constant : Constant
  Constant1 : Constant  Commented=on
  Mux1 : Mux  Inputs=2
  PlantBus : BusSelector  OutputSignals=Vb,alpha,beta,Va,pqr,alphaDot,mach
  PlantBus1 : BusSelector  OutputSignals=Q
  PlantData_1 : InportShadow
  Product : Product
  Product1 : Product
  Scope1 : Scope  Commented=on
  Scope2 : Scope
  Scope3 : Scope
  Scope4 : Scope  Commented=on
  Selector : Selector  Commented=on  InputPortWidth=3  IndexOptions=Index vector (dialog)  Indices=1  OutputSizes=1
  Switch : Switch  Commented=on  Criteria=u2 > Threshold  Threshold=3  SaturateOnIntegerOverflow=off  InputSameDT=off
  nonunit value : Subsystem
  Fb (X Y Z) : Outport  VectorParamsAs1DForOutWhenUnconnected=off
  M (L M N) : Outport  Port=2  VectorParamsAs1DForOutWhenUnconnected=off
  wires:
  "Aerodynamic Forces and Moments "/1 -> Product/1, Scope2/1
  "Aerodynamic Forces and Moments "/2 -> Product1/1, Scope3/1
  PlantData/1 -> PlantBus/1
  Act_surface/1 -> Aerodynamic Coefficients/5(Act_surface)
  PlantBus/2 -> Mux1/1  "<alpha>"
  PlantBus/3 -> Mux1/2  "<beta>"
  PlantBus/5 -> nonunit value/2(pqr)  "<pqr>"
  Center of Gravity/1 -> "Aerodynamic Forces and Moments "/3
  Center of Pressure/1 -> "Aerodynamic Forces and Moments "/4
  PlantBus1/1 -> "Aerodynamic Forces and Moments "/2  "<Q>"
  PlantData_1/1 -> PlantBus1/1
  PlantBus/6 -> nonunit value/3(alphaDot)  "<alphaDot>"
  PlantBus/4 -> nonunit value/1(V)  "<Va>"
  Constant1/1 -> Switch/1
  Constant/1 -> [Aero_SW]
  Switch/1 -> Scope1/1
  Product/1 -> Fb (X Y Z)/1
  Product1/1 -> M (L M N)/1
  [Aero_SW] -> Product/2
  [Aero_SW] -> Product1/2
  PlantBus/1 -> Selector/1  "<Vb>"
  Selector/1 -> Switch/2, Scope4/1  "Vb_x"
  Mux1/1 -> Aerodynamic Coefficients/1(Incid)
  nonunit value/1(pqr_n) -> Aerodynamic Coefficients/3(pqrn)
  nonunit value/2(alphaDot_n) -> Aerodynamic Coefficients/4(alphaDot_n)
  Aerodynamic Coefficients/1(Coeff) -> "Aerodynamic Forces and Moments "/1
  PlantBus/7 -> Aerodynamic Coefficients/2(mach)  "<mach>"

== system eVTOL_PX4_2023b/Subsystem1/airframe1/force moment/gravity in body axis ==
  PlantData : Inport
  EnvmData : Inport  Port=2
  Bus Selector1 : BusSelector  OutputSignals=DCM_be,mass
  Bus Selector2 : BusSelector  OutputSignals=g
  G in body axis : Product  Multiplication=Matrix(*)  RndMeth=Zero
  Gain1 : Gain  Gain=[0; 0; 1]
  Product : Product  RndMeth=Zero
  Fb : Outport  VectorParamsAs1DForOutWhenUnconnected=off
  wires:
  Bus Selector1/1 -> G in body axis/1  "<DCM_be>"
  Gain1/1 -> G in body axis/2
  Bus Selector1/2 -> Product/1  "<mass>"
  Bus Selector2/1 -> Product/2  "<g>"
  Product/1 -> Gain1/1  "mg"
  PlantData/1 -> Bus Selector1/1
  G in body axis/1 -> Fb/1
  EnvmData/1 -> Bus Selector2/1

== system eVTOL_PX4_2023b/Subsystem2/Energy & Power/V_prop1/v_b to v_prop ==
  V_body : Inport
  i : Inport  Port=2
  Add : Sum  Inputs=+-
  Mux1 : Mux  Inputs=2
  Terminator : Terminator
  V_x : Fcn  Expr=u[1]*cos(u[4])
  V_y : Fcn  Expr=0
  V_z : Fcn  Expr=u[3]*sin(u[4])
  V : Outport  VectorParamsAs1DForOutWhenUnconnected=off
  wires:
  i/1 -> Mux1/2
  V_body/1 -> Mux1/1
  Mux1/1 -> V_z/1, V_y/1, V_x/1
  Add/1 -> V/1
  V_x/1 -> Add/1
  V_z/1 -> Add/2
  V_y/1 -> Terminator/1

== system eVTOL_PX4_2023b/Subsystem2/Energy & Power/V_prop2/v_b to v_prop ==
  V_body : Inport
  i : Inport  Port=2
  Add : Sum  Inputs=+-
  Mux1 : Mux  Inputs=2
  Terminator : Terminator
  V_x : Fcn  Expr=u[1]*cos(u[4])
  V_y : Fcn  Expr=0
  V_z : Fcn  Expr=u[3]*sin(u[4])
  V : Outport  VectorParamsAs1DForOutWhenUnconnected=off
  wires:
  i/1 -> Mux1/2
  V_body/1 -> Mux1/1
  Mux1/1 -> V_z/1, V_y/1, V_x/1
  V_z/1 -> Add/2
  V_x/1 -> Add/1
  Add/1 -> V/1
  V_y/1 -> Terminator/1

== system eVTOL_PX4_2023b/Subsystem2/Energy & Power/V_prop3/v_b to v_prop ==
  V_body : Inport
  i : Inport  Port=2
  Add : Sum  Inputs=+-
  Mux1 : Mux  Inputs=2
  Terminator : Terminator
  V_x : Fcn  Expr=u[1]*cos(u[4])
  V_y : Fcn  Expr=0
  V_z : Fcn  Expr=u[3]*sin(u[4])
  V : Outport  VectorParamsAs1DForOutWhenUnconnected=off
  wires:
  i/1 -> Mux1/2
  V_body/1 -> Mux1/1
  Mux1/1 -> V_z/1, V_y/1, V_x/1
  V_z/1 -> Add/2
  V_x/1 -> Add/1
  Add/1 -> V/1
  V_y/1 -> Terminator/1

== system eVTOL_PX4_2023b/Subsystem2/Energy & Power/V_prop4/v_b to v_prop ==
  V_body : Inport
  i : Inport  Port=2
  Add : Sum  Inputs=+-
  Mux1 : Mux  Inputs=2
  Terminator : Terminator
  V_x : Fcn  Expr=u[1]*cos(u[4])
  V_y : Fcn  Expr=0
  V_z : Fcn  Expr=u[3]*sin(u[4])
  V : Outport  VectorParamsAs1DForOutWhenUnconnected=off
  wires:
  i/1 -> Mux1/2
  V_body/1 -> Mux1/1
  Mux1/1 -> V_z/1, V_y/1, V_x/1
  V_x/1 -> Add/1
  Add/1 -> V/1
  V_z/1 -> Add/2
  V_y/1 -> Terminator/1

== system eVTOL_PX4_2023b/Subsystem2/Energy & Power/V_prop5/v_b to v_prop ==
  V_body : Inport
  i : Inport  Port=2
  Add : Sum  Inputs=+-
  Mux1 : Mux  Inputs=2
  Terminator : Terminator
  V_x : Fcn  Expr=u[1]*cos(u[4])
  V_y : Fcn  Expr=0
  V_z : Fcn  Expr=u[3]*sin(u[4])
  V : Outport  VectorParamsAs1DForOutWhenUnconnected=off
  wires:
  i/1 -> Mux1/2
  V_body/1 -> Mux1/1
  Mux1/1 -> V_z/1, V_y/1, V_x/1
  V_z/1 -> Add/2
  V_x/1 -> Add/1
  Add/1 -> V/1
  V_y/1 -> Terminator/1

== system eVTOL_PX4_2023b/Subsystem2/Energy & Power/V_prop6/v_b to v_prop ==
  V_body : Inport
  i : Inport  Port=2
  Add : Sum  Inputs=+-
  Mux1 : Mux  Inputs=2
  Terminator : Terminator
  V_x : Fcn  Expr=u[1]*cos(u[4])
  V_y : Fcn  Expr=0
  V_z : Fcn  Expr=u[3]*sin(u[4])
  V : Outport  VectorParamsAs1DForOutWhenUnconnected=off
  wires:
  i/1 -> Mux1/2
  V_body/1 -> Mux1/1
  Mux1/1 -> V_z/1, V_y/1, V_x/1
  V_z/1 -> Add/2
  V_x/1 -> Add/1
  Add/1 -> V/1
  V_y/1 -> Terminator/1

== system eVTOL_PX4_2023b/Subsystem2/Energy & Power/thrust_1/Motor ==
  P_shaft : Inport
  dt : Inport  Port=2
  V : Inport  Port=3
  rpm0 : Inport  Port=4
  rho : Inport  Port=5
  theta_b : Inport  Port=6
  Add : Sum
  Constant : Constant  Value=Motor.Ue
  Constant1 : Constant  Value=Motor.Re
  Constant2 : Constant  Value=Motor.Rm
  Constant3 : Constant  Value=Motor.KE
  Constant4 : Constant  Value=Motor.KT  VectorParams1D=off
  Constant5 : Constant  Value=Motor.Im0
  Constant6 : Constant  Value=0
  Constant7 : Constant  Value=0.001
  D^5 : Constant  Value=5
  Diameter : Constant  Value=Prop.D
  Diameter1 : Constant  Value=Prop.D
  Divide : Product  Inputs=*//
  Ea : Sum  Inputs=+-
  Gain1 : Gain  Gain=30/pi
  Gain2 : Gain  Gain=pi/30
  Gain3 : Gain  Gain=1/60
  Gain4 : Gain  Gain=1/(2*pi)
  Im : Sum
  Integrator : Integrator  InitialConditionSource=external  InitialCondition=600
  Ix : Constant  Value=Prop.Ix
  J : Product  Inputs=*//
  Manual Switch : ManualSwitch
  Math Function : Math  Operator=magnitude^2  SignedPower=on
  Math Function3 : Math  Operator=pow  SignedPower=on
  Math Function4 : Math  Operator=pow  SignedPower=on
  Memory : Memory  InitialCondition=0.1
  N(rpm) : Product  Inputs=*/
  N(rpm)1 : Product  Inputs=/*
  P Scope : Scope  NumInputPorts=2
  P_sp : Product  Inputs=4
  Product1 : Product
  Product2 : Product
  Q : Product  Inputs=4
  RPM 1 : Scope  NumInputPorts=2
  Saturation : Saturate  UpperLimit=104.72  LowerLimit=0.1
  Scope : Scope
  Sum : Sum  Inputs=|+-
  Ueo : Product
  Um : Sum  Inputs=+-
  get CP : Lookup_n-D  BreakpointsForDimension1=Prop.J  BreakpointsForDimension2=Prop.theta_b  IndexSearchMethod=Linear search  BeginIndexSearchUsingPreviousIndexResult=on  Table=Prop.CP  RndMeth=Simplest
      settings: InputPortMap=u0,u1
  "n^3 " : Constant  Value=3
  rpm : Outport  VectorParamsAs1DForOutWhenUnconnected=off
  wires:
  Saturation/1 -> Gain1/1, Divide/2
  Gain2/1 -> Integrator/2
  rpm0/1 -> Manual Switch/1
  Gain1/1 -> rpm/1, RPM 1/1  "rpm"
  Sum/1 -> Divide/1  "DP"
  Divide/1 -> Integrator/1  "omega_dot"
  Integrator/1 -> Saturation/1  "omega"
  P_sp/1 -> Scope/1, P Scope/1, Sum/1
  P_shaft/1 -> P Scope/2, Sum/2
  Ix/1 -> Divide/3
  Constant/1 -> Ueo/2
  Ueo/1 -> Um/1
  Product1/1 -> Um/2
  Constant1/1 -> Product1/1
  Um/1 -> Ea/1
  Product2/1 -> Ea/2
  Constant2/1 -> Product2/1
  Ea/1 -> N(rpm)/1
  Constant3/1 -> N(rpm)/2
  Diameter/1 -> J/2
  V/1 -> J/1
  N(rpm)/1 -> Gain3/1, RPM 1/2
  J/1 -> get CP/1
  theta_b/1 -> get CP/2
  Gain4/1 -> Q/2  "CQ"
  D^5/1 -> Math Function4/2
  Diameter1/1 -> Math Function4/1
  Math Function/1 -> Q/3  "n^2"
  Q/1 -> N(rpm)1/2
  Constant4/1 -> N(rpm)1/1
  N(rpm)1/1 -> Im/1
  Constant5/1 -> Im/2
  Im/1 -> Product2/2, Product1/2
  rho/1 -> Q/1, P_sp/3  "rho"
  Math Function3/1 -> P_sp/2  "n^3"
  "n^3 "/1 -> Math Function3/2
  Math Function4/1 -> Q/4, P_sp/4  "D^5"
  get CP/1 -> Gain4/1, P_sp/1  "CP"
  Manual Switch/1 -> Gain2/1
  Constant6/1 -> Manual Switch/2
  Constant7/1 -> Add/1
  Add/1 -> Ueo/1
  dt/1 -> Add/2
  Gain3/1 -> Memory/1  "rps"
  Memory/1 -> J/3, Math Function3/1, Math Function/1

== system eVTOL_PX4_2023b/Subsystem2/Energy & Power/thrust_1/Propeller  ==
  rpm : Inport
  V : Inport  Port=2
  rho : Inport  Port=3
  theta_b : Inport  Port=4
  D^5 : Constant  Value=5
  Diameter : Constant  Value=Prop.D
  Display1 : Display
  Display7 : Display
  Divide : Product  Inputs=4
  Divide2 : Product  Inputs=4
  Divide3 : Product  Inputs=**/
  Gain : Gain  Gain=1/60
  Math Function : Math  Operator=magnitude^2  SignedPower=on
  Math Function1 : Math  Operator=magnitude^2  SignedPower=on
  Math Function2 : Math  Operator=magnitude^2  SignedPower=on
  Math Function3 : Math  Operator=pow  SignedPower=on
  Math Function4 : Math  Operator=pow  SignedPower=on
  Scope{,1..4} (5 alike) : Scope
  Subsystem : Subsystem
  get CP : Lookup_n-D  BreakpointsForDimension1=Prop.J  BreakpointsForDimension2=Prop.theta_b  IndexSearchMethod=Linear search  BeginIndexSearchUsingPreviousIndexResult=on  Table=Prop.CP  RndMeth=Simplest
      settings: InputPortMap=u0,u1
  get CT : Lookup_n-D  BreakpointsForDimension1=Prop.J  BreakpointsForDimension2=Prop.theta_b  IndexSearchMethod=Linear search  BeginIndexSearchUsingPreviousIndexResult=on  Table=Prop.CT  RndMeth=Simplest
      settings: InputPortMap=u0,u1
  "n^3 " : Constant  Value=3
  P_plr (w) : Outport  VectorParamsAs1DForOutWhenUnconnected=off
  T (N) : Outport  Port=2  VectorParamsAs1DForOutWhenUnconnected=off
  eta_p : Outport  Port=3  VectorParamsAs1DForOutWhenUnconnected=off
  wires:
  Divide2/1 -> Scope/1, P_plr (w)/1
  Divide3/1 -> eta_p/1  "eta_p"
  D^5/1 -> Math Function4/2
  Math Function4/1 -> Divide2/4
  "n^3 "/1 -> Math Function3/2
  Math Function3/1 -> Divide2/3
  get CP/1 -> Display1/1, Divide3/3, Divide2/1, Scope3/1
  rpm/1 -> Gain/1, Subsystem/2(rpm)
  Subsystem/1(J) -> Scope2/1, get CT/1, Divide3/1, get CP/1
  Divide/1 -> Scope1/1, T (N)/1
  Math Function2/1 -> Divide/4  "D^4"
  Math Function1/1 -> Math Function2/1
  Diameter/1 -> Math Function1/1, Math Function4/1
  Math Function/1 -> Divide/3  "n^2"
  Gain/1 -> Math Function3/1, Math Function/1
  rho/1 -> Divide/2, Divide2/2
  get CT/1 -> Display7/1, Divide3/2, Divide/1, Scope4/1
  V/1 -> Subsystem/1(V)
  theta_b/1 -> get CP/2, get CT/2

== system eVTOL_PX4_2023b/Subsystem2/Energy & Power/thrust_2/Motor ==
  P_shaft : Inport
  dt : Inport  Port=2
  V : Inport  Port=3
  rpm0 : Inport  Port=4
  rho : Inport  Port=5
  theta_b : Inport  Port=6
  Constant : Constant  Value=Motor.Ue
  Constant1 : Constant  Value=Motor.Re
  Constant2 : Constant  Value=Motor.Rm
  Constant3 : Constant  Value=Motor.KE
  Constant4 : Constant  Value=Motor.KT  VectorParams1D=off
  Constant5 : Constant  Value=Motor.Im0
  Constant6 : Constant  Value=0
  D^5 : Constant  Value=5
  Diameter : Constant  Value=Prop.D
  Diameter1 : Constant  Value=Prop.D
  Divide : Product  Inputs=*//
  Ea : Sum  Inputs=+-
  Gain1 : Gain  Gain=30/pi
  Gain2 : Gain  Gain=pi/30
  Gain3 : Gain  Gain=1/60
  Gain4 : Gain  Gain=1/(2*pi)
  Im : Sum
  Integrator : Integrator  InitialConditionSource=external  InitialCondition=600
  Ix : Constant  Value=Prop.Ix
  J : Product  Inputs=*//
  Manual Switch : ManualSwitch
  Math Function : Math  Operator=magnitude^2  SignedPower=on
  Math Function3 : Math  Operator=pow  SignedPower=on
  Math Function4 : Math  Operator=pow  SignedPower=on
  Memory : Memory  InitialCondition=0.1
  N(rpm) : Product  Inputs=*/
  N(rpm)1 : Product  Inputs=/*
  P Scope : Scope  NumInputPorts=2
  P_sp : Product  Inputs=4
  Product1 : Product
  Product2 : Product
  Q : Product  Inputs=4
  RPM 2 : Scope
  Saturation : Saturate  UpperLimit=104.72  LowerLimit=0.1
  Scope : Scope
  Sum : Sum  Inputs=|+-
  Ueo : Product
  Um : Sum  Inputs=+-
  get CP : Lookup_n-D  BreakpointsForDimension1=Prop.J  BreakpointsForDimension2=Prop.theta_b  IndexSearchMethod=Linear search  BeginIndexSearchUsingPreviousIndexResult=on  Table=Prop.CP  RndMeth=Simplest
      settings: InputPortMap=u0,u1
  "n^3 " : Constant  Value=3
  rpm : Outport  VectorParamsAs1DForOutWhenUnconnected=off
  wires:
  Saturation/1 -> Gain1/1, Divide/2
  Gain2/1 -> Integrator/2
  rpm0/1 -> Manual Switch/1
  Gain1/1 -> rpm/1, RPM 2/1  "rpm"
  Sum/1 -> Divide/1  "DP"
  Divide/1 -> Integrator/1  "omega_dot"
  dt/1 -> Ueo/1
  Integrator/1 -> Saturation/1  "omega"
  P_sp/1 -> Scope/1, P Scope/1, Sum/1
  P_shaft/1 -> P Scope/2, Sum/2
  Ix/1 -> Divide/3
  Constant/1 -> Ueo/2
  Ueo/1 -> Um/1
  Product1/1 -> Um/2
  Constant1/1 -> Product1/1
  Um/1 -> Ea/1
  Product2/1 -> Ea/2
  Constant2/1 -> Product2/1
  Ea/1 -> N(rpm)/1
  Constant3/1 -> N(rpm)/2
  Diameter/1 -> J/2
  V/1 -> J/1
  N(rpm)/1 -> Gain3/1
  J/1 -> get CP/1
  theta_b/1 -> get CP/2
  Gain4/1 -> Q/2  "CQ"
  D^5/1 -> Math Function4/2
  Diameter1/1 -> Math Function4/1
  Math Function/1 -> Q/3  "n^2"
  Q/1 -> N(rpm)1/2
  Constant4/1 -> N(rpm)1/1
  N(rpm)1/1 -> Im/1
  Constant5/1 -> Im/2
  Im/1 -> Product2/2, Product1/2
  rho/1 -> Q/1, P_sp/3  "rho"
  Math Function3/1 -> P_sp/2  "n^3"
  "n^3 "/1 -> Math Function3/2
  Math Function4/1 -> Q/4, P_sp/4  "D^5"
  get CP/1 -> Gain4/1, P_sp/1  "CP"
  Constant6/1 -> Manual Switch/2
  Manual Switch/1 -> Gain2/1
  Gain3/1 -> Memory/1  "rps"
  Memory/1 -> J/3, Math Function3/1, Math Function/1
